simulink model "Simulink_1"  (R2013b)
settings: Solver=ode45  StartTime=0.0  StopTime=50.0  RelTol=1e-5
settings Model: Creator=99900361  LastModifiedBy=99900361
settings DataIOCC: SignalLoggingSaveFormat=ModelDataLogs  SignalLoggingName=sigsOut
settings DebuggingCC: SaveWithParameterizedLinksMsg=none  SignalResolutionControl=TryResolveAllWithWarning  SolverPrmCheckMsg=none  MultiTaskDSMMsg=warning  MultiTaskCondExecSysMsg=none  StrictBusMsg=None
settings HardwareCC: TargetUnknown=on
settings RTWCC: IncludeERTFirstTime=on
settings GRTTargetCC: CombineOutputUpdateFcns=off  GRTInterface=on

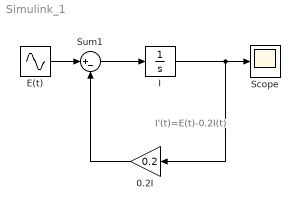
== system Simulink_1 ==
  note: I'(t)=E(t)-0.2I(t)
  0.2I : Gain  Gain=0.2  SaturateOnIntegerOverflow=on  OutDataTypeStr=Inherit: Same as input  ParamDataTypeStr=Inherit: Same as input
  E(t) : Sin  Amplitude=5  SampleTime=0
  I : Integrator
  Scope : Scope
  Sum1 : Sum  Inputs=|+-  SaturateOnIntegerOverflow=on
  wires:
  E(t)/1 -> Sum1/1
  Sum1/1 -> I/1
  I/1 -> Scope/1, 0.2I/1
  0.2I/1 -> Sum1/2
